simulink model "sgMdl_IO191_AnalogDigitalLoopback"  (R2024b)
settings: Solver=FixedStepAuto  StartTime=0.0  StopTime=inf  RelTol=1e-3  EnableMultiTasking=on
undefined symbols (not defined in the file): Ended, Single
libraries: speedgoatlib_IO191 x5
Description:
  | IO191 - Analog and Digital Loopback
settings Model: ModifiedByFormat=Speedgoat  SimulationMode=external  ExtModeTrigDuration=100000  Creator=Speedgoat  LastModifiedBy=Speedgoat
settings SolverCC: ConcurrentTasks=on  AlgebraicLoopSolver=TrustRegion  PositivePriorityOrder=on
settings DataIOCC: LimitDataPoints=on  SaveFormat=StructureWithTime  ReturnWorkspaceOutputs=off
settings OptimizationCC: BlockReduction=off  OptimizeBlockIOStorage=off  BufferReuse=off  GlobalBufferReuse=off  ExpressionFolding=off  LocalBlockOutputs=off  OptimizeDataStoreBuffers=off  BusAssignmentInplaceUpdate=off
settings DebuggingCC: TasksWithSamePriorityMsg=none  UnconnectedInputMsg=warning  UnconnectedOutputMsg=warning  UnconnectedLineMsg=warning  AllowSymbolicDim=off  SFUnexpectedBacktrackingDiag=warning  SFNoUnconditionalDefaultTransitionDiag=warning  ArithmeticOperatorsInVariantConditions=warning
settings HardwareCC: ProdBitPerLong=64  ProdLongLongMode=on  ProdHWDeviceType=Intel->x86-64 (Linux 64)
settings ModelReferenceCC: EnableRefExpFcnMdlSchedulingChecks=on  PropagateSignalLabelsOutOfModel=off
settings SFSimCC: SimUseLocalCustomCode=off  CustomCodeUndefinedFunction=UseInterfaceOnly
settings RTWCC: Description=Speedgoat Real-Time Target Machine  SystemTargetFile=speedgoat.tlc  TemplateMakefile=slrealtime_default_tmf  RTWUseLocalCustomCode=off  Toolchain=Simulink Real-Time Toolchain  BuildConfiguration=Faster Runs  TargetLang=C++  GPUComputeCapability=3.5  DLArmComputeVersion=19.05
settings CodeAppCC: StateflowObjectComments=on
settings SimulinkRealTimeTargetCC: SubcomponentCodeInterfacePackaging=Reusable function  InstructionSetFMA=off  LogToMDFFile=off  SLRTFileLogMaxRuns=10  UseGCCFastMath=on
settings ConfigComp: CovMetricSettings=dw  CovSaveCumulativeToWorkspaceVar=on  CovSaveSingleToWorkspaceVar=on  CovExternalEMLEnable=off  CovBoundaryAbsTol=1.0e-5

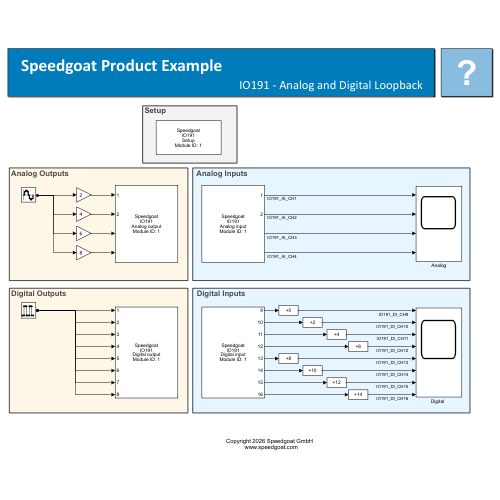
[thumbnail: Simulink's stored preview of the top-level diagram]
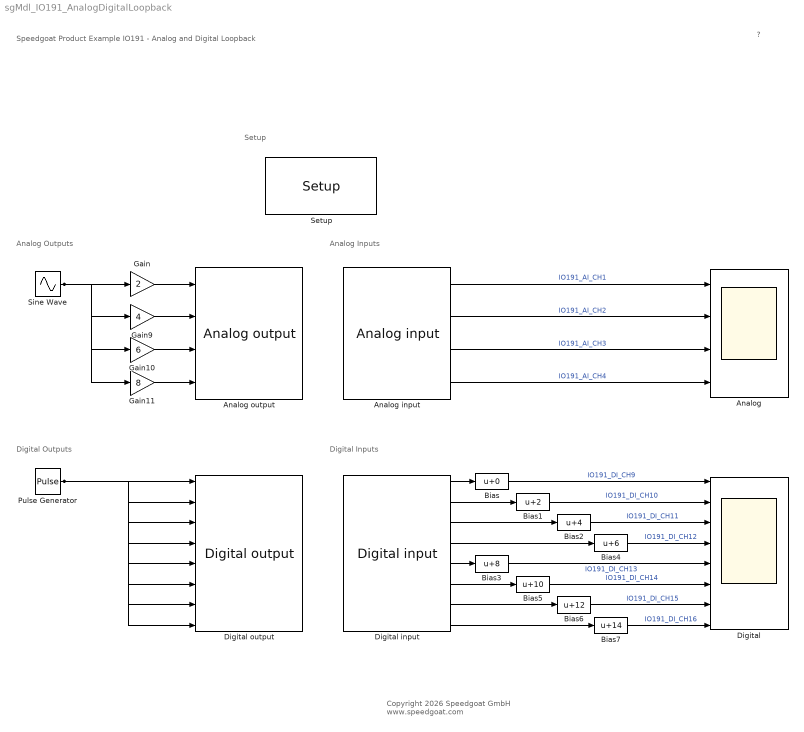
== system sgMdl_IO191_AnalogDigitalLoopback ==
  note: Digital Outputs
  note: Digital Inputs
  note: Setup
  note: Analog Outputs
  note: Analog Inputs
  note: Speedgoat Product Example
      | IO191 - Analog and Digital Loopback
  note: ?
  note: Copyright 2026 Speedgoat GmbH
      |  www.speedgoat.com
  Analog : Scope  NumInputPorts=4
  "Analog input " : speedgoatlib_IO191/Analog input   parModuleId=1  parSampleTime=0.001  parPciSlot=-1  parAdcChannels=[1 2 3 4]  parAdcMode=2  parAdcRanges=[3 3 3 3]  parAdcInitValues=[0 0]  parAdcResets=[1 1]  paramsAdcDma=[0 1 200 -1]
      settings: SourceProductName=Simulink Real-Time: Speedgoat I/O Blockset
  "Analog output " : speedgoatlib_IO191/Analog output   parModuleId=1  parSampleTime=0.001  parPciSlot=-1  parDacChannels=[1 2 3 4]  parModuleType=1  parDacRanges=[4 4 4 4]  parDacInitValues=[0 0 0 0]  parDacResets=[1 1 1 1]
      settings: SourceProductName=Simulink Real-Time: Speedgoat I/O Blockset
  Bias : Bias  SaturateOnIntegerOverflow=off
  Bias1 : Bias  Bias=2  SaturateOnIntegerOverflow=off
  Bias2 : Bias  Bias=4  SaturateOnIntegerOverflow=off
  Bias3 : Bias  Bias=8  SaturateOnIntegerOverflow=off
  Bias4 : Bias  Bias=6  SaturateOnIntegerOverflow=off
  Bias5 : Bias  Bias=10  SaturateOnIntegerOverflow=off
  Bias6 : Bias  Bias=12  SaturateOnIntegerOverflow=off
  Bias7 : Bias  Bias=14  SaturateOnIntegerOverflow=off
  "Digital  " : Scope  NumInputPorts=8
  "Digital input " : speedgoatlib_IO191/Digital input   parModuleId=1  parSampleTime=0.001  parPortConf=Separate port for each active input channel  parDataType=Double  parPciSlot=-1  parDiChannels=[9 10 11 12 13 14 15 16]
      settings: SourceProductName=Simulink Real-Time: Speedgoat I/O Blockset
  "Digital output " : speedgoatlib_IO191/Digital output   parModuleId=1  parSampleTime=0.001  parPortConf=Separate port for each active output channel  parPciSlot=-1  parDoChannels=[1 2 3 4 5 6 7 8]  parDoInitValues=[0 0 0 0 0 0 0 0]  parDoResets=[1 1 1 1 1 1 1 1]
      settings: SourceProductName=Simulink Real-Time: Speedgoat I/O Blockset
  Gain : Gain  Gain=2
  Gain10 : Gain  Gain=6
  Gain11 : Gain  Gain=8
  Gain9 : Gain  Gain=4
  Pulse Generator : DiscretePulseGenerator  Period=20  PulseWidth=10  SampleTime=0.001
  "Setup " : speedgoatlib_IO191/Setup   parModuleId=1  parPciSlot=-1  parTriggerSignal=TTL  parAdcChannels=[1 2 3 4]  parAdcRanges=[3 3 3 3]  parAdcChannel1=on  parAdcChannel2=on  parAdcChannel3=on  parAdcChannel4=on  parAdcChannel5=off  parAdcChannel6=off  parAdcChannel7=off  parAdcChannel8=off  parAdcMode=Single-Ended  parAdcRange11=+-10.24 V  parAdcRange21=+-24.576 V  parAdcRange12=+-10.24 V  parAdcRange22=+-24.576 V  parAdcRange13=+-10.24 V  parAdcRange23=+-24.576 V  parAdcRange14=+-10.24 V  parAdcRange24=+-24.576 V  parAdcRange15=+-10.24 V  parAdcRange25=+-24.576 V  parAdcRange16=+-10.24 V  parAdcRange26=+-24.576 V  parAdcRange17=+-10.24 V  parAdcRange27=+-24.576 V  parAdcRange18=+-10.24 V  parAdcRange28=+-24.576 V  parAdcEnDma=off  parAdcFrame=125  parAdcDiv=200  parAdcSample=-1  parDacChannels=[1 2 3 4]  parDacChannel1=on  parDacChannel2=on  parDacChannel3=on  parDacChannel4=on  parDacMode=Single-Ended  parDacRanges=[4 4 4 4]  parDacInitValues=[0 0 0 0]  parDacResets=[1 1 1 1]  parDacRange1=+-10 V  parDacInitValue1=0  parDacReset1=on  parDacRange2=+-10 V  parDacInitValue2=0  parDacReset2=on  parDacRange3=+-10 V  parDacInitValue3=0  parDacReset3=on  parDacRange4=+-10 V  parDacInitValue4=0  parDacReset4=on  parDiChannels=[9 10 11 12 13 14 15 16]  parDoChannels=[1 2 3 4 5 6 7 8]  parDioFirstControl=1  parDioSecondControl=0  parDioChannel1=Out  parExtra1=I  parExtra2=I  parExtra3=I  parDioChannel2=In  parDioChannel3=In  parDioChannel4=In  parDioChannel5=In  parDioChannel6=In  parDioChannel7=In  parDioChannel8=In  parDioChannel9=In  parDoInitValues=[0 0 0 0]  parDoResets=[1 1 1 1]  parDoInitValue1=0  parDoReset1=on  parDoInitValue2=0  parDoReset2=on  parDoInitValue3=0  parDoReset3=on  parDoInitValue4=0  parDoReset4=on  parDoInitValue5=0  parDoReset5=on  parDoInitValue6=0  parDoReset6=on  parDoInitValue7=0  parDoReset7=on  parDoInitValue8=0  parDoReset8=on  parDoInitValue9=0  parDoReset9=on  parDoInitValue10=0  parDoReset10=on  parDoInitValue11=0  parDoReset11=on  parDoInitValue12=0  parDoReset12=on  parDoInitValue13=0  parDoReset13=on  parDoInitValue14=0  parDoReset14=on  parDoInitValue15=0  parDoReset15=on  parDoInitValue16=0  parDoReset16=on
      settings: SourceProductName=Simulink Real-Time: Speedgoat I/O Blockset
  Sine Wave : Sin  Frequency=2*pi  SampleTime=0.001
  wires:
  Pulse Generator/1 -> "Digital output "/8, "Digital output "/7, "Digital output "/6, "Digital output "/5, "Digital output "/4, "Digital output "/3, "Digital output "/2, "Digital output "/1
  "Analog input "/1 -> Analog/1  "IO191_AI_CH1"
  "Analog input "/2 -> Analog/2  "IO191_AI_CH2"
  "Analog input "/3 -> Analog/3  "IO191_AI_CH3"
  "Analog input "/4 -> Analog/4  "IO191_AI_CH4"
  Gain11/1 -> "Analog output "/4
  Sine Wave/1 -> Gain11/1, Gain10/1, Gain9/1, Gain/1
  Gain10/1 -> "Analog output "/3
  Gain9/1 -> "Analog output "/2
  Gain/1 -> "Analog output "/1
  "Digital input "/7 -> Bias6/1
  "Digital input "/3 -> Bias2/1
  "Digital input "/4 -> Bias4/1
  "Digital input "/5 -> Bias3/1
  "Digital input "/6 -> Bias5/1
  Bias1/1 -> "Digital  "/2  "IO191_DI_CH10"
  "Digital input "/1 -> Bias/1
  Bias6/1 -> "Digital  "/7  "IO191_DI_CH15"
  Bias7/1 -> "Digital  "/8  "IO191_DI_CH16"
  Bias3/1 -> "Digital  "/5  "IO191_DI_CH13"
  Bias5/1 -> "Digital  "/6  "IO191_DI_CH14"
  "Digital input "/2 -> Bias1/1
  Bias4/1 -> "Digital  "/4  "IO191_DI_CH12"
  Bias2/1 -> "Digital  "/3  "IO191_DI_CH11"
  Bias/1 -> "Digital  "/1  "IO191_DI_CH9"
  "Digital input "/8 -> Bias7/1
